simulink model "tire_model_experimental"  (R2016a)
settings: Solver=VariableStepAuto  StartTime=0.0  StopTime=10.0  RelTol=1e-3
values from neighbouring files (symbols this model uses):
  C_alpha = 120000    [dynamics.m]    (also in setup.m; tire_test.m = 197)
  mu = 0.37    [dynamics.m]    (also in setup.m; tire_test.m = 1.31)
settings Model: Creator=Cyrus  LastModifiedBy=Cyrus

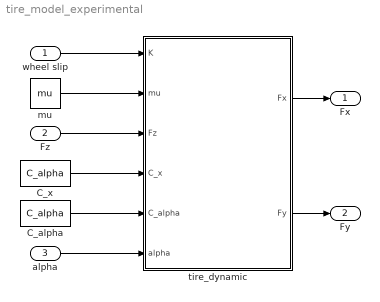
== system tire_model_experimental ==
  wheel slip : Inport
  Fz : Inport  Port=2
  alpha : Inport  Port=3
  C_alpha : Constant  Value=C_alpha
  C_x : Constant  Value=C_alpha
  mu : Constant  Value=mu
  tire_dynamic : MATLAB Function  TreatAsAtomicUnit=on
  Fx : Outport
  Fy : Outport  Port=2
  wires:
  mu/1 -> tire_dynamic/2(mu)
  Fz/1 -> tire_dynamic/3(Fz)
  C_alpha/1 -> tire_dynamic/5(C_alpha)
  alpha/1 -> tire_dynamic/6(alpha)
  C_x/1 -> tire_dynamic/4(C_x)
  tire_dynamic/2(Fy) -> Fy/1
  tire_dynamic/1(Fx) -> Fx/1
  wheel slip/1 -> tire_dynamic/1(K)

== matlab function tire_model_experimental/tire_dynamic ==
  data: K input; Fx output; mu input; Fz input; C_x input; C_alpha input; Fy output; alpha input
function [Fx, Fy] = fcn(K, mu, Fz, C_x, C_alpha, alpha)
%#codegen
    if K == -1
        K = -0.99;
    end
 
    gamma = sqrt(C_x^2*(K/(1+K))^2+C_alpha^2*(tan(alpha)/(1+K))^2);
    
    if gamma <= 3*mu*Fz
        F = gamma - 1/(3*mu*Fz)*gamma^2 + 1/(27*mu^2*Fz^2)*gamma^3;
    else
        F = mu*Fz;
    end
    
    if gamma == 0
        Fx = 0;
        Fy = 0;
    else
        Fx = C_x/gamma * (K/(1+K)) * F;
        Fy = -C_alpha/gamma * (tan(alpha)/(1+K)) * F;
    end
end
